simulink model "untitled"  (R2023a)
settings: Solver=VariableStepAuto  StartTime=0.0  StopTime=10.0  RelTol=1e-3
values from neighbouring files (symbols this model uses):
  e = 0    [orb_elem.m]
  mi = (mi)    [orb_elem.m]
undefined symbols (not defined in the file or in its folder): Cd0, Cd1, drag, h0_ini, i0_ini, J2, J2_dist, l0, l1, m0, m1, man, ohm0_ini, omega_E, pcoRad, r0_dot_ini, r0_ini, Re, theta0_ini, x0_dot_ini, x0_ini, y0_dot_ini, y0_ini, z0_dot_ini, z0_ini
(part 1 of 2)
settings Model: Creator=rodri  LastModifiedBy=rodri

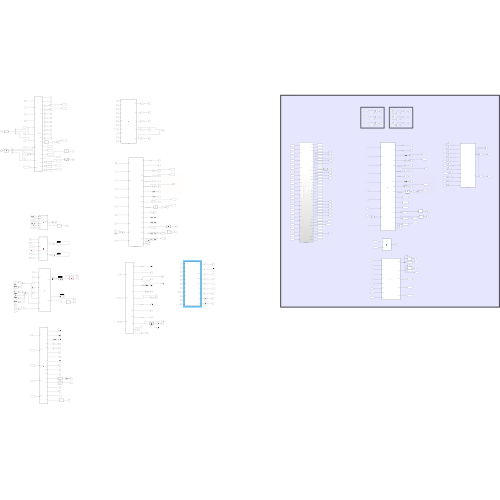
[thumbnail: Simulink's stored preview of the top-level diagram]
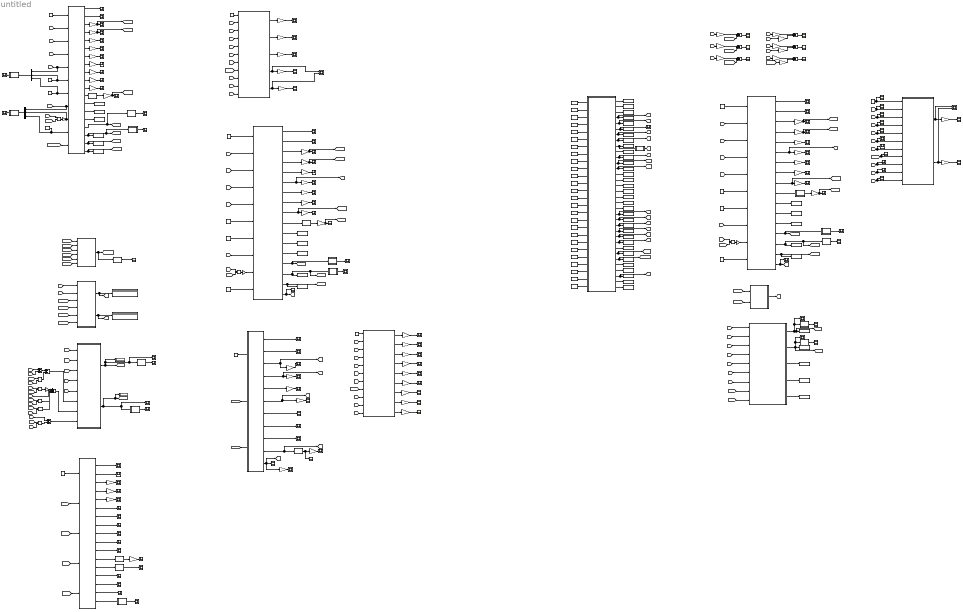
== system untitled ==
  note: Diferença elementos orbitais do líder e do seguidor
  note: Diferença elementos orbitais do líder e do seguidor
  note: Diferença elementos orbitais do líder entre o integral e o calculado
  Add : Sum
  Add1 : Sum  Inputs=+-
  Add2 : Sum  Inputs=+++-
  Add3 : Sum
  Constant{1,6,8,15,36} (5 alike) : Constant  Value=mi
  Constant{3..5,7,9..11,13..14,33,45..46} (12 alike) : Constant  Value=0
  Constant12 : Constant  Value=Re
  Constant2 : Constant  Value=Re
  Constant34 : Constant  Value=r0_dot_ini
  Constant35 : Constant  Value=Re
  Constant37 : Constant  Value=theta0_ini
  Constant41 : Constant  Value=ohm0_ini
  Constant42 : Constant  Value=e  LockScale=on
  Constant43 : Constant  Value=m1
  Constant44 : Constant  Value=J2_dist  OutDataTypeStr=boolean
  Constant47 : Constant  Value=x0_ini
  Constant48 : Constant  Value=Cd1
  Constant49 : Constant  Value=m0
  Constant50 : Constant  Value=y0_ini
  Constant51 : Constant  Value=z0_ini
  Constant52 : Constant  Value=x0_dot_ini
  Constant53 : Constant  Value=y0_dot_ini
  Constant54 : Constant  Value=z0_dot_ini
  Constant55 : Constant  Value=man
  Constant56 : Constant  Value=pcoRad
  Constant57 : Constant  Value=l1
  Constant58 : Constant  Value=l0
  Constant59 : Constant  Value=r0_ini
  Constant60 : Constant  Value=Cd0
  Constant61 : Constant  Value=drag  OutDataTypeStr=boolean
  Constant62 : Constant  Value=h0_ini
  Constant63 : Constant  Value=i0_ini
  Display{,1..3} (4 alike) : Display
  ElemOrbLider : MATLAB Function  TreatAsAtomicUnit=on
  ElemOrbLider1 : MATLAB Function  TreatAsAtomicUnit=on
  ElemOrbLider2 : MATLAB Function  TreatAsAtomicUnit=on
  Gain{,1..9,12..28,30..43,45..64} (61 alike) : Gain  Gain=180/pi
  Gain{10..11,29,44} (4 alike) : Gain
  GuiamentoOrbital1 : Subsystem
  MATLAB Function : MATLAB Function  TreatAsAtomicUnit=on
  MATLAB Function1 : MATLAB Function  TreatAsAtomicUnit=on
  MATLAB Function10 : MATLAB Function  TreatAsAtomicUnit=on
  MATLAB Function11 : MATLAB Function  TreatAsAtomicUnit=on
  MATLAB Function12 : MATLAB Function  TreatAsAtomicUnit=on
  MATLAB Function13 : MATLAB Function  TreatAsAtomicUnit=on
  MATLAB Function14 : MATLAB Function  TreatAsAtomicUnit=on
  MATLAB Function15 : MATLAB Function  TreatAsAtomicUnit=on
  MATLAB Function16 : MATLAB Function  TreatAsAtomicUnit=on
  MATLAB Function17 : MATLAB Function  TreatAsAtomicUnit=on
  MATLAB Function18 : MATLAB Function  TreatAsAtomicUnit=on
  MATLAB Function19 : MATLAB Function  TreatAsAtomicUnit=on
  MATLAB Function2 : MATLAB Function  TreatAsAtomicUnit=on
  MATLAB Function3 : MATLAB Function  TreatAsAtomicUnit=on
  MATLAB Function4 : MATLAB Function  TreatAsAtomicUnit=on
  MATLAB Function5 : MATLAB Function  TreatAsAtomicUnit=on
  MATLAB Function6 : MATLAB Function  TreatAsAtomicUnit=on
  MATLAB Function7 : MATLAB Function  TreatAsAtomicUnit=on
  MATLAB Function8 : MATLAB Function  TreatAsAtomicUnit=on
  MATLAB Function9 : MATLAB Function  TreatAsAtomicUnit=on
  Minus{,1..5} (6 alike) : Sum  Inputs=+-
  Mux2 : Mux  Inputs=3
  Mux3 : Mux  Inputs=3
  Nadir1 : MATLAB Function  TreatAsAtomicUnit=on
  Nadir2 : MATLAB Function  TreatAsAtomicUnit=on
  Nadir3 : MATLAB Function  TreatAsAtomicUnit=on
  OrbEleSeg : MATLAB Function  TreatAsAtomicUnit=on
  OrbEleSeg1 : MATLAB Function  TreatAsAtomicUnit=on
  Product{,1..7} (8 alike) : Product
  Scope{,1..74,76..103,105..116} (115 alike) : Scope
  Scope104 : Scope  NumInputPorts=2
  Scope75 : Scope  NumInputPorts=2
  To Workspace1 : ToWorkspace  VariableName=r0x_vec_I1  SaveFormat=Timeseries  SampleTime=-1
  To Workspace10 : ToWorkspace  VariableName=h0_vec_I2  SaveFormat=Timeseries  SampleTime=-1
  To Workspace11 : ToWorkspace  VariableName=r0x_vec_I2  SaveFormat=Timeseries  SampleTime=-1
  To Workspace12 : ToWorkspace  VariableName=v0_vec_I2  SaveFormat=Timeseries  SampleTime=-1
  To Workspace13 : ToWorkspace  VariableName=r0y_vec_I2  SaveFormat=Timeseries  SampleTime=-1
  To Workspace14 : ToWorkspace  VariableName=v1_vec_I  SaveFormat=Timeseries  SampleTime=-1
  To Workspace15 : ToWorkspace  VariableName=r1x_vec_I  SaveFormat=Timeseries  SampleTime=-1
  To Workspace16 : ToWorkspace  VariableName=r1y_vec_I  SaveFormat=Timeseries  SampleTime=-1
  To Workspace17 : ToWorkspace  VariableName=r1z_vec_I  SaveFormat=Timeseries  SampleTime=-1
  To Workspace18 : ToWorkspace  VariableName=r0z_vec_I2  SaveFormat=Timeseries  SampleTime=-1
  To Workspace2 : ToWorkspace  VariableName=r0x_vec_I  SaveFormat=Timeseries  SampleTime=-1
  To Workspace28 : ToWorkspace  VariableName=v0_vec_I  SaveFormat=Timeseries  SampleTime=-1
  To Workspace3 : ToWorkspace  VariableName=r0y_vec_I  SaveFormat=Timeseries  SampleTime=-1
  To Workspace34 : ToWorkspace  VariableName=x_dotdot  SaveFormat=Timeseries  SampleTime=-1
  To Workspace35 : ToWorkspace  VariableName=y_dotdot  SaveFormat=Timeseries  SampleTime=-1
  To Workspace36 : ToWorkspace  VariableName=ohm0  SaveFormat=Timeseries  SampleTime=-1
  To Workspace37 : ToWorkspace  VariableName=omega_x  SaveFormat=Timeseries  SampleTime=-1
  To Workspace38 : ToWorkspace  VariableName=omega_z  SaveFormat=Timeseries  SampleTime=-1
  To Workspace39 : ToWorkspace  VariableName=dx0  SaveFormat=Timeseries  SampleTime=-1
  To Workspace4 : ToWorkspace  VariableName=r0z_vec_I  SaveFormat=Timeseries  SampleTime=-1
  To Workspace40 : ToWorkspace  VariableName=dy0  SaveFormat=Timeseries  SampleTime=-1
  To Workspace41 : ToWorkspace  VariableName=dz0  SaveFormat=Timeseries  SampleTime=-1
  To Workspace45 : ToWorkspace  VariableName=a0_vec_I  SaveFormat=Timeseries  SampleTime=-1
  To Workspace46 : ToWorkspace  VariableName=h0_vec_I  SaveFormat=Timeseries  SampleTime=-1
  To Workspace47 : ToWorkspace  VariableName=delta_Dx  SaveFormat=Timeseries  SampleTime=-1
  To Workspace48 : ToWorkspace  VariableName=delta_Dy  SaveFormat=Timeseries  SampleTime=-1
  To Workspace49 : ToWorkspace  VariableName=delta_Dz  SaveFormat=Timeseries  SampleTime=-1
  To Workspace5 : ToWorkspace  VariableName=v0_vec_I1  SaveFormat=Timeseries  SampleTime=-1
  To Workspace50 : ToWorkspace  VariableName=rho_a0  SaveFormat=Timeseries  SampleTime=-1
  To Workspace51 : ToWorkspace  VariableName=z_dotdot  SaveFormat=Timeseries  SampleTime=-1
  To Workspace52 : ToWorkspace  VariableName=x  SaveFormat=Timeseries  SampleTime=-1
  To Workspace53 : ToWorkspace  VariableName=x_dot  SaveFormat=Timeseries  SampleTime=-1
  To Workspace54 : ToWorkspace  VariableName=y  SaveFormat=Timeseries  SampleTime=-1
  To Workspace55 : ToWorkspace  VariableName=y_dot  SaveFormat=Timeseries  SampleTime=-1
  To Workspace56 : ToWorkspace  VariableName=z  SaveFormat=Timeseries  SampleTime=-1
  To Workspace57 : ToWorkspace  VariableName=z_dot  SaveFormat=Timeseries  SampleTime=-1
  To Workspace58 : ToWorkspace  VariableName=rho_a1  SaveFormat=Timeseries  SampleTime=-1
  To Workspace59 : ToWorkspace  VariableName=r0_dotdot  SaveFormat=Timeseries  SampleTime=-1
  To Workspace6 : ToWorkspace  VariableName=r0y_vec_I1  SaveFormat=Timeseries  SampleTime=-1
  To Workspace60 : ToWorkspace  VariableName=omega_z_dot  SaveFormat=Timeseries  SampleTime=-1
  To Workspace61 : ToWorkspace  VariableName=dx1  SaveFormat=Timeseries  SampleTime=-1
  To Workspace62 : ToWorkspace  VariableName=r0  SaveFormat=Timeseries  SampleTime=-1
  To Workspace63 : ToWorkspace  VariableName=dy1  SaveFormat=Timeseries  SampleTime=-1
  To Workspace64 : ToWorkspace  VariableName=dz1  SaveFormat=Timeseries  SampleTime=-1
  To Workspace65 : ToWorkspace  VariableName=omega_y_dot  SaveFormat=Timeseries  SampleTime=-1
  To Workspace66 : ToWorkspace  VariableName=omega_x_dot  SaveFormat=Timeseries  SampleTime=-1
  To Workspace67 : ToWorkspace  VariableName=h0  SaveFormat=Timeseries  SampleTime=-1
  To Workspace68 : ToWorkspace  VariableName=r1  SaveFormat=Timeseries  SampleTime=-1
  To Workspace69 : ToWorkspace  VariableName=r0_dot  SaveFormat=Timeseries  SampleTime=-1
  To Workspace7 : ToWorkspace  VariableName=r0z_vec_I1  SaveFormat=Timeseries  SampleTime=-1
  To Workspace70 : ToWorkspace  VariableName=i0  SaveFormat=Timeseries  SampleTime=-1
  To Workspace71 : ToWorkspace  VariableName=theta0  SaveFormat=Timeseries  SampleTime=-1
  To Workspace72 : ToWorkspace  VariableName=theta0_dot  SaveFormat=Timeseries  SampleTime=-1
  To Workspace8 : ToWorkspace  VariableName=h0_vec_I1  SaveFormat=Timeseries  SampleTime=-1
  To Workspace9 : ToWorkspace  VariableName=r1_vec_I  SaveFormat=Timeseries  SampleTime=-1
  wrapTo2pi1 : MATLAB Function  TreatAsAtomicUnit=on
  wrapTo2pi2 : MATLAB Function  TreatAsAtomicUnit=on
  wrapTo2pi3 : MATLAB Function  TreatAsAtomicUnit=on
  wrapTo2pi4 : MATLAB Function  TreatAsAtomicUnit=on
  wrapTo2pi5 : MATLAB Function  TreatAsAtomicUnit=on
  wrapTo2pi6 : MATLAB Function  TreatAsAtomicUnit=on
  wires:
  Product/1 -> Gain11/1
  Constant8/1 -> ElemOrbLider/1(mi)
  Gain10/1 -> Add2/1
  [v0_vec_I] -> OrbEleSeg/5(v0_vec_I)
  [z] -> Product4/2
  [x] -> Product3/2
  Add1/1 -> MATLAB Function5/6(x_dot)
  [r0_dot] -> Add/1
  ElemOrbLider/6(f1) -> Gain3/1
  Mux2/1 -> MATLAB Function14/1(u)
  Constant7/1 -> Mux2/3, ElemOrbLider/7(z)
  Add/1 -> Add1/1
  ElemOrbLider/2(e1) -> Scope1/1
  [h0_vec_I] -> MATLAB Function3/6(h0_vec_I)
  OrbEleSeg/7(u1) -> Scope63/1
  ElemOrbLider/5(omega1) -> Gain2/1
  [r0_vec_I] -> OrbEleSeg/4(r0_vec_I)
  [z] -> MATLAB Function5/5(z)
  OrbEleSeg/5(omega1) -> Gain41/1
  OrbEleSeg/17(v1_vec_I) -> MATLAB Function10/1(x)
  MATLAB Function16/1(rho) -> Scope30/1
  Gain41/1 -> Scope61/1
  MATLAB Function9/1(rho) -> Scope78/1
  MATLAB Function6/1(y) -> Scope72/1
  MATLAB Function8/1(rho) -> Scope77/1
  ElemOrbLider/15(r0z_I) -> To Workspace4/1
  OrbEleSeg/4(Ohm1) -> Gain40/1
  [h0] -> MATLAB Function3/2(h0)
  OrbEleSeg/10(omega_t1) -> Scope66/1
  OrbEleSeg/3(i1) -> Gain39/1
  [rho_vec_I] -> OrbEleSeg/2(rho_vec_I)
  Gain40/1 -> Scope60/1
  Gain42/1 -> Scope68/1
  Constant36/1 -> OrbEleSeg/1(mi)
  [y] -> MATLAB Function5/4(y)
  [omega_z] -> MATLAB Function/2(omega_z)
  [r0_dotdot_vec] -> ElemOrbLider/11(r0_dotdot_vec)
  Gain39/1 -> Scope59/1
  OrbEleSeg/11(lambda1) -> Scope67/1
  OrbEleSeg/12(theta1) -> wrapTo2pi3/1(u)
  [omega_z_dot] -> MATLAB Function/4(omega_z_dot)
  MATLAB Function14/1(y) -> Scope24/1
  [omega_x] -> MATLAB Function/6(omega_x)
  [a0_vec_I] -> MATLAB Function3/5(a0_vec_I)
  [omega_x] -> Product4/1
  ElemOrbLider/19(h0_vec_I) -> [h0_vec_I], To Workspace46/1
  wrapTo2pi3/1(y) -> Gain42/1
  [C_dot] -> MATLAB Function5/2(C_dot)
  [C] -> MATLAB Function5/1(C)
  ElemOrbLider/18(a0_vec_I) -> [a0_vec_I], To Workspace45/1
  [r0_dot] -> MATLAB Function/5(r0_dot)
  Gain4/1 -> [theta0_calc], Scope6/1
  [r0_dotdot] -> MATLAB Function/1(r0_dotdot)
  OrbEleSeg/8(L1) -> Scope64/1
  ElemOrbLider/11(lambda1) -> Gain9/1
  [ohm0] -> ElemOrbLider/2(ohm)
  Gain3/1 -> Scope5/1
  ElemOrbLider/3(i1) -> Gain/1
  Gain2/1 -> Scope4/1
  Gain/1 -> [i0_calc], Scope2/1
  Gain5/1 -> Scope7/1
  Gain6/1 -> Scope8/1
  [theta0] -> ElemOrbLider/3(theta)
  ElemOrbLider/12(theta1) -> wrapTo2pi2/1(u)
  [r0] -> Product/1
  ElemOrbLider/8(L1) -> Gain6/1
  ElemOrbLider/16(r0_vec_I) -> MATLAB Function7/1(x), [r0_vec_I]
  ElemOrbLider/1(a1) -> Scope/1
  Product4/1 -> Add2/4
  [omega_z] -> Product3/1
  ElemOrbLider/13(r0x_I) -> To Workspace2/1
  MATLAB Function3/2(C_dot) -> [C_dot], Display1/1
  OrbEleSeg/2(e1) -> Scope58/1
  [r0] -> MATLAB Function3/1(r0)
  Product1/1 -> Add1/2
  [r0_dot] -> Mux3/1, ElemOrbLider/8(x_dot)
  MATLAB Function15/1(y) -> Scope25/1
  [x_dot] -> Add/2
  OrbEleSeg/9(l1) -> Scope65/1
  [y] -> Product5/2
  Product5/1 -> Add3/2
  ElemOrbLider/17(v0_vec_I) -> MATLAB Function8/1(x), [v0_vec_I], To Workspace28/1
  ElemOrbLider/7(u1) -> Gain5/1
  [omega_z] -> Product1/1
  Gain7/1 -> Scope9/1
  OrbEleSeg/16(r1z_I) -> Scope12/1
  [omega_z] -> Product2/2
  [y_dot] -> Add2/2
  ElemOrbLider/9(l1) -> Gain7/1
  OrbEleSeg/1(a1) -> Scope57/1
  Constant9/1 -> ElemOrbLider/10(z_dot), Mux3/3
  Gain11/1 -> Mux3/2, ElemOrbLider/9(y_dot)
  [x] -> MATLAB Function5/3(x)
  MATLAB Function5/2(rho_dot_vec_I) -> [rho_dot_vec_I], Display3/1, Scope27/1, MATLAB Function16/1(x)
  MATLAB Function3/1(C) -> Display/1, [C]
  ElemOrbLider/14(r0y_I) -> To Workspace3/1
  ElemOrbLider/10(omega_t1) -> Gain8/1
  MATLAB Function5/1(rho_vec_I) -> Scope26/1, MATLAB Function17/1(x), Display2/1, [rho_vec_I]
  ElemOrbLider/4(Ohm1) -> Gain1/1
  [z_dot] -> Add3/1
  [i0] -> ElemOrbLider/4(I)
  Product2/1 -> Gain10/1
  MATLAB Function17/1(rho) -> Scope29/1
  [r0] -> Product2/1
  wrapTo2pi2/1(y) -> Gain4/1
  OrbEleSeg/13(r1_vec_I) -> MATLAB Function9/1(x)
  [r0] -> MATLAB Function/3(r0)
  [omega_z] -> Product/2
  OrbEleSeg/14(r1x_I) -> Scope14/1
  MATLAB Function/1(r0_dotdot_vec) -> MATLAB Function6/1(u), [r0_dotdot_vec]
  OrbEleSeg/15(r1y_I) -> Scope13/1
  [omega_x] -> Product5/1
  Gain9/1 -> Scope11/1
  [rho_dot_vec_I] -> OrbEleSeg/3(rho_dot_vec_I)
  [y] -> Product1/2
  Add3/1 -> MATLAB Function5/8(z_dot)
  Mux3/1 -> MATLAB Function15/1(u)
  Constant5/1 -> Mux2/2, ElemOrbLider/6(y)
  OrbEleSeg/6(f1) -> Scope62/1
  MATLAB Function10/1(rho) -> Scope79/1
  Gain1/1 -> [ohm0_calc], Scope3/1
  MATLAB Function7/1(rho) -> Scope76/1
  [r0_vec_I] -> MATLAB Function3/3(r0_vec_I)
  Add2/1 -> MATLAB Function5/7(y_dot)
  Product3/1 -> Add2/3
  [r0] -> Mux2/1, ElemOrbLider/5(x)
  Gain8/1 -> Scope10/1
  [v0_vec_I] -> MATLAB Function3/4(v0_vec_I)
  Gain50/1 -> Scope44/1
  [i0] -> Nadir2/7(i0)
  [ohm1] -> Nadir2/9(ohm1)
  [y] -> Nadir2/4(y)
  Constant35/1 -> Nadir2/1(Re)
  Gain51/1 -> Scope42/1
  [z] -> Nadir2/5(z)
  [ohm0] -> Nadir2/6(ohm0)
  [r0] -> Nadir2/2(r0)
  Nadir2/4(PHI) -> Scope75/1, Gain52/1
  Gain53/1 -> Scope74/1
  [i1] -> Nadir2/10(i1)
  Gain52/1 -> Scope73/1
  Nadir2/3(LF1) -> Gain51/1
  [x] -> Nadir2/3(x)
  [L0] -> Nadir2/8(f0)
  [L1] -> Nadir2/11(f1)
  Nadir2/5(THETA) -> Scope75/2, Gain53/1
  Nadir2/2(psi_ref) -> Gain50/1  "psi_ref"
  Nadir2/1(phi_ref) -> Gain49/1  "phi_ref"
  Gain49/1 -> Scope43/1
  Nadir1/3(alpha_F1) -> Gain12/1
  OrbEleSeg1/6(f1) -> [f1], Gain25/1  "Anomalia verdadeira"
  wrapTo2pi4/1(y) -> Scope16/1, Gain16/1
  Gain21/1 -> Scope32/1
  Gain18/1 -> Scope21/1
  Gain17/1 -> Scope20/1
  OrbEleSeg1/4(Ohm1) -> [ohm1], Gain14/1  "Longitude do nodo ascendente"
  Nadir1/1(LF1) -> Gain24/1
  OrbEleSeg1/10(theta1) -> [theta1], wrapTo2pi4/1(u)  "Argumento de latitude"
  [z] -> Nadir1/5(z)
  Gain13/1 -> Scope34/1
  Nadir1/5(alpha_f) -> Gain18/1
  [ohm0] -> Nadir1/6(ohm0)
  OrbEleSeg1/9(lambda1) -> Scope40/1  "Longitude média"
  Gain14/1 -> Scope36/1
  OrbEleSeg1/3(i1) -> [i1], Gain13/1  "inclinação"
  OrbEleSeg1/2(e1) -> Scope23/1  "excentricidade"
  Gain15/1 -> Scope37/1
  Gain22/1 -> Scope33/1
  Nadir1/8(psi_ref) -> Gain21/1
  Gain16/1 -> Scope41/1
  Gain19/1 -> Scope28/1
  OrbEleSeg1/1(a1) -> Scope22/1  "semi-eixo maior"
  OrbEleSeg1/7(l1) -> Scope38/1  "Latitude média"
  [i0] -> Nadir1/7(i0)
  Constant1/1 -> OrbEleSeg1/1(mi)
  [L1] -> Nadir1/8(L0)
  Constant2/1 -> Nadir1/1(Re)
  [v1_vec_I] -> OrbEleSeg1/3(v1_vec_I)
  [L1] -> Nadir1/11(L1)
  Nadir1/9(phi_ref) -> Gain22/1
  Nadir1/7(THETA) -> Gain20/1
  [ohm1] -> Nadir1/9(ohm1)
  Gain12/1 -> Scope19/1
  OrbEleSeg1/8(omega_t1) -> Scope39/1  "Longitude do pericentro"
  [i1] -> Nadir1/10(i1)
  [x] -> Nadir1/3(x)
  [r0] -> Nadir1/2(r0)
  Gain23/1 -> Scope35/1
  Gain26/1 -> Scope18/1
  [y] -> Nadir1/4(y)
  Gain24/1 -> Scope45/1
  Nadir1/6(PHI) -> Gain19/1
  OrbEleSeg1/11(L1) -> [L1], Gain26/1, Scope17/1
  Nadir1/2(LF2) -> Gain23/1
  [r1_vec_I] -> OrbEleSeg1/2(r1_vec_I)
  OrbEleSeg1/5(omega1) -> Gain15/1  "Argumento do pericentro"
  Gain25/1 -> Scope15/1
  Gain20/1 -> Scope31/1
  Nadir1/4(alpha_F2) -> Gain17/1
  [theta0] -> ElemOrbLider1/3(theta)
  ElemOrbLider1/3(i0) -> Gain27/1  "inclinação"
  ElemOrbLider1/15(v0_vec_I) -> To Workspace5/1, MATLAB Function2/1(x), [v0_vec_I]
  Product6/1 -> Gain29/1
  Constant10/1 -> ElemOrbLider1/10(z_dot)
  Constant4/1 -> ElemOrbLider1/7(z)
  ElemOrbLider1/2(e0) -> Scope47/1  "excentricidade"
  Gain30/1 -> Scope51/1
  Gain35/1 -> Scope70/1
  [r0] -> Product6/1
  [ohm0] -> ElemOrbLider1/2(ohm)
  ElemOrbLider1/1(a0) -> Scope46/1  "semi-eixo maior"
  ElemOrbLider1/5(omega0) -> Gain30/1  "Argumento do pericentro"
  Gain32/1 -> [theta0_calc], Scope53/1
  Gain34/1 -> Scope69/1
  ElemOrbLider1/9(lambda0) -> [lambda0], Gain35/1  "Longitude média"
  Gain31/1 -> Scope52/1
  [r0_dot] -> ElemOrbLider1/8(x_dot)
  ElemOrbLider1/12(r0y_I) -> To Workspace6/1
  [omega_z] -> Product6/2
  MATLAB Function2/1(rho) -> Scope56/1
  ElemOrbLider1/10(theta0) -> wrapTo2pi1/1(u)  "Argumento de latitude"
  ElemOrbLider1/6(f0) -> [f0], Gain31/1  "Anomalia verdadeira"
  ElemOrbLider1/16(h0_vec_I) -> To Workspace8/1, [h0_vec_I]
  wrapTo2pi1/1(y) -> Gain32/1
  Gain33/1 -> Scope54/1
  MATLAB Function1/1(rho) -> Scope55/1
  Gain29/1 -> ElemOrbLider1/9(y_dot)
  ElemOrbLider1/4(Ohm0) -> Gain28/1  "Longitude do nodo ascendente"
  ElemOrbLider1/13(r0z_I) -> To Workspace7/1
  Gain28/1 -> [ohm0_calc], Scope50/1
  Constant6/1 -> ElemOrbLider1/1(mi)
  ElemOrbLider1/17(L0) -> [L0], Scope48/1
  ElemOrbLider1/14(r0_vec_I) -> [r0_vec_I], MATLAB Function1/1(x)
  ElemOrbLider1/7(l0) -> Gain33/1  "Latitude média"
  Gain27/1 -> [i0_calc], Scope49/1
  ElemOrbLider1/8(omega_t0) -> Gain34/1  "Longitude do perigeu"
  Constant3/1 -> ElemOrbLider1/6(y)
  [i0] -> ElemOrbLider1/4(I)
  ElemOrbLider1/11(r0x_I) -> To Workspace1/1
  [r0] -> ElemOrbLider1/5(x)
  [r0] -> Scope90/1, Nadir3/2(r0)  "r0"
  Constant60/1 -> GuiamentoOrbital1/3(Cd0)
  GuiamentoOrbital1/18(delta_Dy) -> To Workspace48/1
  Minus/1 -> Scope108/1
  [y] -> Scope92/1, Nadir3/4(y)  "y"
  GuiamentoOrbital1/16(dz0) -> To Workspace41/1
  [i1] -> Scope101/1, Nadir3/10(i1)  "i1"
  MATLAB Function11/1(y) -> Scope84/1
  [i0] -> Scope96/1, Nadir3/7(i0)  "i0"
  GuiamentoOrbital1/31(dy1) -> To Workspace63/1
  [z] -> Scope94/1, Nadir3/5(z)  "z"
  Nadir3/1(AZ) -> Scope104/1, Gain46/1  "AZ"
  [ohm0] -> Scope95/1, Nadir3/6(ohm0)  "ohm0"
  Minus5/1 -> Scope114/1
  [x] -> Scope91/1, Nadir3/3(x)  "x"
  [L0] -> Scope99/1, Nadir3/8(L0)  "L0"
  Nadir3/2(EL) -> Scope104/2, Gain45/1  "EL"
  Minus2/1 -> Scope109/1
  MATLAB Function4/2(v1_vec_I) -> [v1_vec_I], Scope83/1, MATLAB Function13/1(u), To Workspace14/1
  [ohm1] -> Scope100/1, Nadir3/9(ohm1)  "ohm1"
  [r0_vec_I] -> MATLAB Function4/8(r0_vec_I)
  Constant48/1 -> GuiamentoOrbital1/5(Cd1)
  Constant53/1 -> GuiamentoOrbital1/17(y0_dot_ini)
  Constant52/1 -> GuiamentoOrbital1/16(x0_dot_ini)
  Gain46/1 -> Scope98/1
  MATLAB Function4/3(r1x_vec_I) -> To Workspace15/1
  MATLAB Function13/1(y) -> Scope85/1
  GuiamentoOrbital1/27(rho_a1) -> To Workspace58/1
  Constant41/1 -> GuiamentoOrbital1/12(ohm0_ini)
  wrapTo2pi5/1(y) -> [theta0]
  Constant44/1 -> GuiamentoOrbital1/23(J2_dist)
  [z_dot] -> MATLAB Function4/7(z_dot)
  Constant58/1 -> GuiamentoOrbital1/2(l0)
  [C] -> MATLAB Function4/1(C)
  [x] -> MATLAB Function4/2(x)
  Minus3/1 -> Scope113/1
  [z] -> MATLAB Function4/4(z)
  [i1] -> Gain62/1
  [v0_vec_I] -> MATLAB Function4/9(v0_vec_I)
  [x_dot] -> MATLAB Function4/5(x_dot)
  [y_dot] -> MATLAB Function4/6(y_dot)
  Constant61/1 -> GuiamentoOrbital1/21(drag)
  GuiamentoOrbital1/6(r1) -> Scope89/1, To Workspace68/1
  [theta1] -> Gain64/1
  Constant47/1 -> GuiamentoOrbital1/13(x0_ini)
  Gain45/1 -> Scope97/1
  GuiamentoOrbital1/20(rho_a0) -> To Workspace50/1
  Constant54/1 -> GuiamentoOrbital1/18(z0_dot_ini)
  Constant59/1 -> GuiamentoOrbital1/8(r0_ini)
  GuiamentoOrbital1/19(delta_Dz) -> To Workspace49/1
  Constant56/1 -> GuiamentoOrbital1/20(pcoRad)
  Gain59/1 -> Minus3/1
  [ohm0] -> Gain60/1
  Gain57/1 -> Minus1/1
  GuiamentoOrbital1/11(ohm0) -> [ohm0], To Workspace36/1
  [theta0] -> Gain61/1
  Gain62/1 -> Minus3/2
  Gain58/1 -> Minus2/1
  MATLAB Function12/1(C) -> [C]
  [i0] -> Gain59/1
  [r0_vec_I] -> MATLAB Function12/1(r0_vec_I)
  [h0_vec_I] -> MATLAB Function12/2(h0_vec_I)
  Gain64/1 -> Minus5/2
  Gain61/1 -> Minus5/1
  Minus1/1 -> Scope107/1
  [i0_calc] -> Minus/2
  [ohm0_calc] -> Minus1/2
  GuiamentoOrbital1/8(i0) -> [i0], To Workspace70/1
  Constant55/1 -> GuiamentoOrbital1/19(man)
  GuiamentoOrbital1/24(y_dot) -> [y_dot], To Workspace55/1
  [y] -> MATLAB Function4/3(y)
  MATLAB Function4/5(r1z_vec_I) -> To Workspace17/1
  Constant43/1 -> GuiamentoOrbital1/4(m1)
  GuiamentoOrbital1/21(x) -> [x], To Workspace52/1
  GuiamentoOrbital1/30(dx1) -> To Workspace61/1
  GuiamentoOrbital1/10(theta0_dot) -> To Workspace72/1
  Minus4/1 -> Scope111/1
  Constant45/1 -> GuiamentoOrbital1/25(uy)
  GuiamentoOrbital1/13(omega_z) -> [omega_z], To Workspace38/1
  Constant57/1 -> GuiamentoOrbital1/6(l1)
  Constant46/1 -> GuiamentoOrbital1/26(uz)
  GuiamentoOrbital1/3(z_dotdot) -> To Workspace51/1
  GuiamentoOrbital1/28(r0_dotdot) -> [r0_dotdot], To Workspace59/1
  GuiamentoOrbital1/12(omega_x) -> [omega_x], To Workspace37/1
  [theta0] -> Gain58/1
  MATLAB Function4/4(r1y_vec_I) -> To Workspace16/1
  GuiamentoOrbital1/22(x_dot) -> [x_dot], To Workspace53/1
  Constant34/1 -> GuiamentoOrbital1/7(r0_dot_ini)
  Gain63/1 -> Minus4/2
  GuiamentoOrbital1/34(omega_x_dot) -> To Workspace66/1
  Constant50/1 -> GuiamentoOrbital1/14(y0_ini)
  Gain56/1 -> Minus/1
  GuiamentoOrbital1/26(z_dot) -> [z_dot], To Workspace57/1
  GuiamentoOrbital1/15(dy0) -> To Workspace40/1
  GuiamentoOrbital1/25(z) -> [z], To Workspace56/1
  GuiamentoOrbital1/9(theta0) -> wrapTo2pi5/1(u), To Workspace71/1
  GuiamentoOrbital1/5(h0) -> [h0], To Workspace67/1
  Constant63/1 -> GuiamentoOrbital1/10(i0_ini)
  [i0] -> Gain56/1
  GuiamentoOrbital1/32(dz1) -> [dz1], To Workspace64/1
  GuiamentoOrbital1/23(y) -> [y], To Workspace54/1
  GuiamentoOrbital1/4(r0) -> [r0], To Workspace62/1
  GuiamentoOrbital1/2(y_dotdot) -> To Workspace35/1
  GuiamentoOrbital1/33(omega_y_dot) -> To Workspace65/1
  GuiamentoOrbital1/7(r0_dot) -> [r0_dot], To Workspace69/1
  MATLAB Function4/1(r1_vec_I) -> [r1_vec_I], To Workspace9/1, Scope82/1, MATLAB Function11/1(u)
  GuiamentoOrbital1/29(omega_z_dot) -> [omega_z_dot], To Workspace60/1
  ElemOrbLider2/11(r0x_I) -> To Workspace11/1
  Constant42/1 -> GuiamentoOrbital1/22(e)
  [r0_dot] -> ElemOrbLider2/8(x_dot)
  [ohm0] -> Gain57/1
  Gain43/1 -> [ohm0_calc], Scope102/1
  [r0] -> Product7/1
  wrapTo2pi6/1(y) -> Gain47/1
  ElemOrbLider2/12(r0y_I) -> To Workspace13/1
  Gain60/1 -> Minus4/1
  ElemOrbLider2/8(omega_t0) -> Gain54/1  "Longitude do perigeu"
  Constant37/1 -> GuiamentoOrbital1/11(theta0_ini)
  [theta0] -> ElemOrbLider2/3(theta)
  Gain38/1 -> [i0_calc], Scope93/1
  Constant14/1 -> ElemOrbLider2/7(z)
  ElemOrbLider2/3(i0) -> Gain38/1  "inclinação"
  [ohm0] -> ElemOrbLider2/2(ohm)
  [L1] -> Scope103/1, Nadir3/11(L1)  "L1"
  Constant13/1 -> ElemOrbLider2/6(y)
  Gain37/1 -> Scope105/1
  ElemOrbLider2/15(v0_vec_I) -> To Workspace12/1, MATLAB Function19/1(x), [v0_vec_I]
  ElemOrbLider2/2(e0) -> Scope86/1  "excentricidade"
  Gain54/1 -> Scope80/1
  ElemOrbLider2/1(a0) -> Scope71/1  "semi-eixo maior"
  ElemOrbLider2/14(r0_vec_I) -> [r0_vec_I], MATLAB Function18/1(x)
  Constant49/1 -> GuiamentoOrbital1/1(m0)
  Gain36/1 -> Scope110/1
  Gain55/1 -> Scope81/1
  GuiamentoOrbital1/17(delta_Dx) -> To Workspace47/1
  [ohm1] -> Gain63/1
  GuiamentoOrbital1/1(x_dotdot) -> To Workspace34/1
  ElemOrbLider2/9(lambda0) -> [lambda0], Gain55/1  "Longitude média"
  ElemOrbLider2/16(h0_vec_I) -> To Workspace10/1, [h0_vec_I]
  MATLAB Function18/1(rho) -> Scope115/1
  [omega_z] -> Product7/2
  ElemOrbLider2/13(r0z_I) -> To Workspace18/1
  Constant62/1 -> GuiamentoOrbital1/9(h0_ini)
  ElemOrbLider2/7(l0) -> Gain48/1  "Latitude média"
  MATLAB Function19/1(rho) -> Scope116/1
  Product7/1 -> Gain44/1
  ElemOrbLider2/6(f0) -> [f0], Gain37/1  "Anomalia verdadeira"
  Gain44/1 -> ElemOrbLider2/9(y_dot)
  Constant12/1 -> Scope88/1, Nadir3/1(Re)  "Re"
  Gain48/1 -> Scope112/1
  Constant33/1 -> GuiamentoOrbital1/24(ux)
  Constant15/1 -> ElemOrbLider2/1(mi)
  ElemOrbLider2/4(Ohm0) -> Gain43/1  "Longitude do nodo ascendente"
  GuiamentoOrbital1/14(dx0) -> To Workspace39/1
  Constant11/1 -> ElemOrbLider2/10(z_dot)
  Constant51/1 -> GuiamentoOrbital1/15(z0_ini)
  [r0] -> ElemOrbLider2/5(x)
  Gain47/1 -> [theta0_calc], Scope106/1
  ElemOrbLider2/5(omega0) -> Gain36/1  "Argumento do pericentro"
  [i0] -> ElemOrbLider2/4(I)
  [theta0_calc] -> Minus2/2
  ElemOrbLider2/10(theta0) -> wrapTo2pi6/1(u)  "Argumento de latitude"
  ElemOrbLider2/17(L0) -> [L0], Scope87/1

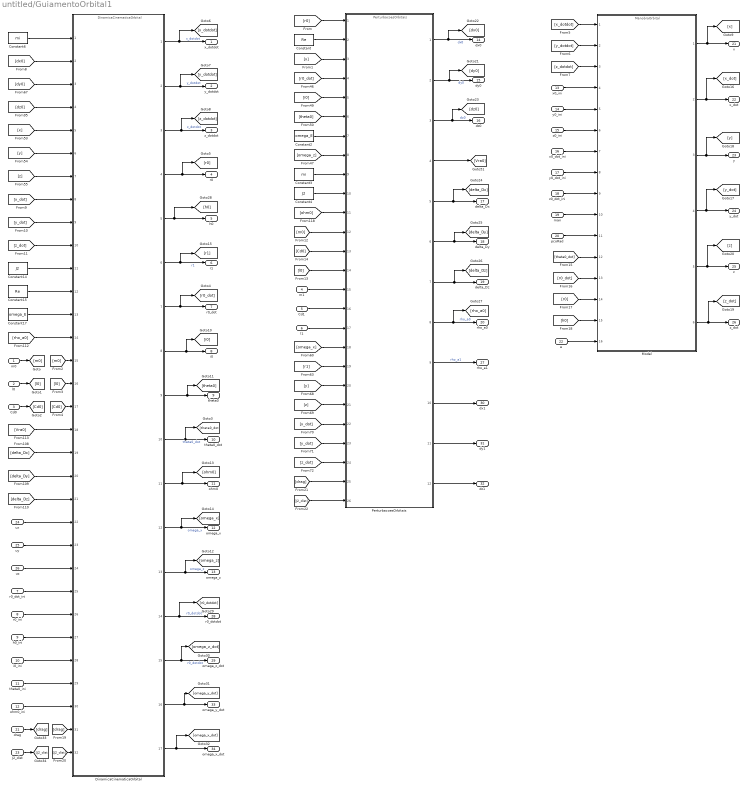
== system untitled/GuiamentoOrbital1 ==
  m0 : Inport  OutDataTypeStr=double  PortDimensions=1
  l0 : Inport  Port=2  OutDataTypeStr=double  PortDimensions=1
  Cd0 : Inport  Port=3  OutDataTypeStr=double  PortDimensions=1
  m1 : Inport  Port=4  OutDataTypeStr=double  PortDimensions=1
  Cd1 : Inport  Port=5  OutDataTypeStr=double  PortDimensions=1
  l1 : Inport  Port=6  OutDataTypeStr=double  PortDimensions=1
  r0_dot_ini : Inport  Port=7  OutDataTypeStr=double  PortDimensions=1
  r0_ini : Inport  Port=8  OutDataTypeStr=double  PortDimensions=1
  h0_ini : Inport  Port=9  OutDataTypeStr=double  PortDimensions=1
  i0_ini : Inport  Port=10  OutDataTypeStr=double  PortDimensions=1
  theta0_ini : Inport  Port=11  OutDataTypeStr=double  PortDimensions=1
  ohm0_ini : Inport  Port=12  OutDataTypeStr=double  PortDimensions=1
  x0_ini : Inport  Port=13  OutDataTypeStr=double  PortDimensions=1
  y0_ini : Inport  Port=14  OutDataTypeStr=double  PortDimensions=1
  z0_ini : Inport  Port=15  OutDataTypeStr=double  PortDimensions=1
  x0_dot_ini : Inport  Port=16  OutDataTypeStr=double  PortDimensions=1
  y0_dot_ini : Inport  Port=17  OutDataTypeStr=double  PortDimensions=1
  z0_dot_ini : Inport  Port=18  OutDataTypeStr=double  PortDimensions=1
  man : Inport  Port=19  OutDataTypeStr=boolean  PortDimensions=1
  pcoRad : Inport  Port=20  OutDataTypeStr=double  PortDimensions=1
  drag : Inport  Port=21  OutDataTypeStr=boolean  PortDimensions=1
  e : Inport  Port=22  OutDataTypeStr=double  PortDimensions=1
  J2_dist : Inport  Port=23  OutDataTypeStr=boolean  PortDimensions=1
  ux : Inport  Port=24  OutDataTypeStr=double  PortDimensions=1
  uy : Inport  Port=25  OutDataTypeStr=double  PortDimensions=1
  uz : Inport  Port=26  OutDataTypeStr=double  PortDimensions=1
  Constant : Constant  Value=Re
  Constant14 : Constant  Value=J2
  Constant15 : Constant  Value=Re
  Constant17 : Constant  Value=omega_E
  Constant2 : Constant  Value=omega_E
  Constant3 : Constant  Value=mi
  Constant4 : Constant  Value=J2
  Constant6 : Constant  Value=mi
  DinamicaCinematicaOrbital : ModelReference  ModelNameDialog=DinamicaCinematicaOrbital  ModelReferenceVersion=3.29
  Model : ModelReference  ModelNameDialog=ManobraOrbital.slx  ModelReferenceVersion=3.34
  PerturbacoesOrbitais : ModelReference  ModelNameDialog=PerturbacoesOrbitais  ModelReferenceVersion=3.14
  x_dotdot : Outport  OutDataTypeStr=double  PortDimensions=1  SampleTime=0
  y_dotdot : Outport  Port=2  OutDataTypeStr=double  PortDimensions=1  SampleTime=0
  z_dotdot : Outport  Port=3  OutDataTypeStr=double  PortDimensions=1  SampleTime=0
  r0 : Outport  Port=4  OutDataTypeStr=double  PortDimensions=1  SampleTime=0
  h0 : Outport  Port=5  OutDataTypeStr=double  PortDimensions=1  SampleTime=0
  r1 : Outport  Port=6  OutDataTypeStr=double  PortDimensions=1  SampleTime=0
  r0_dot : Outport  Port=7  OutDataTypeStr=double  PortDimensions=1  SampleTime=0
  i0 : Outport  Port=8  OutDataTypeStr=double  PortDimensions=1  SampleTime=0
  theta0 : Outport  Port=9  OutDataTypeStr=double  PortDimensions=1  SampleTime=0
  theta0_dot : Outport  Port=10  OutDataTypeStr=double  PortDimensions=1  SampleTime=0
  ohm0 : Outport  Port=11  OutDataTypeStr=double  PortDimensions=1  SampleTime=0
  omega_x : Outport  Port=12  OutDataTypeStr=double  PortDimensions=1  SampleTime=0
  omega_z : Outport  Port=13  OutDataTypeStr=double  PortDimensions=1  SampleTime=0
  dx0 : Outport  Port=14  OutDataTypeStr=double  PortDimensions=1  SampleTime=[1,0]
  dy0 : Outport  Port=15  OutDataTypeStr=double  PortDimensions=1  SampleTime=[1,0]
  dz0 : Outport  Port=16  OutDataTypeStr=double  PortDimensions=1  SampleTime=[1,0]
  delta_Dx : Outport  Port=17  OutDataTypeStr=double  PortDimensions=1  SampleTime=[1,0]
  delta_Dy : Outport  Port=18  OutDataTypeStr=double  PortDimensions=1  SampleTime=[1,0]
  delta_Dz : Outport  Port=19  OutDataTypeStr=double  PortDimensions=1  SampleTime=[1,0]
  rho_a0 : Outport  Port=20  OutDataTypeStr=double  PortDimensions=1  SampleTime=[1,0]
  x : Outport  Port=21  OutDataTypeStr=double  PortDimensions=1  SampleTime=0
  x_dot : Outport  Port=22  OutDataTypeStr=double  PortDimensions=1  SampleTime=0
  y : Outport  Port=23  OutDataTypeStr=double  PortDimensions=1  SampleTime=0
  y_dot : Outport  Port=24  OutDataTypeStr=double  PortDimensions=1  SampleTime=0
  z : Outport  Port=25  OutDataTypeStr=double  PortDimensions=1  SampleTime=0
  z_dot : Outport  Port=26  OutDataTypeStr=double  PortDimensions=1  SampleTime=0
  rho_a1 : Outport  Port=27  OutDataTypeStr=double  PortDimensions=1  SampleTime=[1,0]
  r0_dotdot : Outport  Port=28  OutDataTypeStr=double  PortDimensions=1  SampleTime=0
  omega_z_dot : Outport  Port=29  OutDataTypeStr=double  PortDimensions=1  SampleTime=0
  dx1 : Outport  Port=30  OutDataTypeStr=double  PortDimensions=1  SampleTime=[1,0]
  dy1 : Outport  Port=31  OutDataTypeStr=double  PortDimensions=1  SampleTime=[1,0]
  dz1 : Outport  Port=32  OutDataTypeStr=double  PortDimensions=1  SampleTime=[1,0]
  omega_y_dot : Outport  Port=33  OutDataTypeStr=double  PortDimensions=1  SampleTime=0
  omega_x_dot : Outport  Port=34  OutDataTypeStr=double  PortDimensions=1  SampleTime=0
  wires:
  DinamicaCinematicaOrbital/6 -> r1/1, [r1]  "r1"
  PerturbacoesOrbitais/4 -> [Vra0]
  x0_dot_ini/1 -> Model/7
  DinamicaCinematicaOrbital/8 -> i0/1, [i0]
  DinamicaCinematicaOrbital/12 -> omega_x/1, [omega_x]  "omega_x"
  man/1 -> Model/10
  DinamicaCinematicaOrbital/10 -> [theta0_dot], theta0_dot/1  "theta0_dot"
  [Cd0] -> DinamicaCinematicaOrbital/17
  uz/1 -> DinamicaCinematicaOrbital/24
  [z] -> DinamicaCinematicaOrbital/7
  [Cd0] -> PerturbacoesOrbitais/13
  e/1 -> Model/16
  PerturbacoesOrbitais/9 -> rho_a1/1  "rho_a1"
  r0_ini/1 -> DinamicaCinematicaOrbital/26
  [rho_a0] -> DinamicaCinematicaOrbital/14
  [h0] -> Model/15
  [i0] -> PerturbacoesOrbitais/5
  Cd0/1 -> [Cd0]
  uy/1 -> DinamicaCinematicaOrbital/23
  [r0] -> PerturbacoesOrbitais/1
  i0_ini/1 -> DinamicaCinematicaOrbital/28
  Constant14/1 -> DinamicaCinematicaOrbital/11
  [theta0_dot] -> Model/12
  [x_dot] -> PerturbacoesOrbitais/22
  m1/1 -> PerturbacoesOrbitais/15
  theta0_ini/1 -> DinamicaCinematicaOrbital/29
  Cd1/1 -> PerturbacoesOrbitais/16
  l0/1 -> [l0]
  l1/1 -> PerturbacoesOrbitais/17
  m0/1 -> [m0]
  [m0] -> PerturbacoesOrbitais/12
  [l0] -> DinamicaCinematicaOrbital/16
  [m0] -> DinamicaCinematicaOrbital/15
  [z_dot] -> DinamicaCinematicaOrbital/10
  [y] -> DinamicaCinematicaOrbital/6
  [dy0] -> DinamicaCinematicaOrbital/3
  [y_dot] -> DinamicaCinematicaOrbital/9
  [r0] -> Model/14
  [delta_Dz] -> DinamicaCinematicaOrbital/21
  Constant15/1 -> DinamicaCinematicaOrbital/12
  PerturbacoesOrbitais/7 -> delta_Dz/1, [delta_Dz]
  [x_dot] -> DinamicaCinematicaOrbital/8
  [dz0] -> DinamicaCinematicaOrbital/4
  [x] -> DinamicaCinematicaOrbital/5
  DinamicaCinematicaOrbital/1 -> x_dotdot/1, [x_dotdot]  "x_dotdot"
  Constant3/1 -> PerturbacoesOrbitais/9
  [dx0] -> DinamicaCinematicaOrbital/2
  PerturbacoesOrbitais/2 -> [dy0], dy0/1  "dy0"
  [delta_Dx] -> DinamicaCinematicaOrbital/19
  r0_dot_ini/1 -> DinamicaCinematicaOrbital/25
  h0_ini/1 -> DinamicaCinematicaOrbital/27
  [x] -> PerturbacoesOrbitais/3
  DinamicaCinematicaOrbital/9 -> theta0/1, [theta0]
  [z_dotdot] -> Model/3
  [z] -> PerturbacoesOrbitais/21
  [Vra0] -> DinamicaCinematicaOrbital/18
  [l0] -> PerturbacoesOrbitais/14
  [r0_dot] -> PerturbacoesOrbitais/4
  PerturbacoesOrbitais/6 -> delta_Dy/1, [delta_Dy]
  ohm0_ini/1 -> DinamicaCinematicaOrbital/30
  ux/1 -> DinamicaCinematicaOrbital/22
  PerturbacoesOrbitais/1 -> dx0/1, [dx0]  "dx0"
  Constant/1 -> PerturbacoesOrbitais/2
  Model/5 -> z/1, [z]
  [y] -> PerturbacoesOrbitais/20
  Model/4 -> y_dot/1, [y_dot]
  Constant6/1 -> DinamicaCinematicaOrbital/1
  [z_dot] -> PerturbacoesOrbitais/24
  Model/1 -> x/1, [x]
  Model/3 -> y/1, [y]
  Constant4/1 -> PerturbacoesOrbitais/10
  PerturbacoesOrbitais/3 -> dz0/1, [dz0]  "dz0"
  DinamicaCinematicaOrbital/7 -> [r0_dot], r0_dot/1
  [y_dot] -> PerturbacoesOrbitais/23
  PerturbacoesOrbitais/8 -> [rho_a0], rho_a0/1  "rho_a0"
  Constant17/1 -> DinamicaCinematicaOrbital/13
  DinamicaCinematicaOrbital/5 -> [h0], h0/1
  [ohm0] -> PerturbacoesOrbitais/11
  Constant2/1 -> PerturbacoesOrbitais/7
  DinamicaCinematicaOrbital/13 -> [omega_z], omega_z/1  "omega_z"
  DinamicaCinematicaOrbital/3 -> [z_dotdot], z_dotdot/1  "z_dotdot"
  DinamicaCinematicaOrbital/2 -> [y_dotdot], y_dotdot/1  "y_dotdot"
  DinamicaCinematicaOrbital/4 -> [r0], r0/1
  [delta_Dy] -> DinamicaCinematicaOrbital/20
  Model/6 -> z_dot/1, [z_dot]
  y0_dot_ini/1 -> Model/8
  DinamicaCinematicaOrbital/11 -> [ohm0], ohm0/1
  pcoRad/1 -> Model/11
  [omega_z] -> PerturbacoesOrbitais/8
  [theta0] -> PerturbacoesOrbitais/6
  [r0_dot] -> Model/13
  [omega_x] -> PerturbacoesOrbitais/18
  y0_ini/1 -> Model/5
  [x_dotdot] -> Model/1
  x0_ini/1 -> Model/4
  [r1] -> PerturbacoesOrbitais/19
  z0_dot_ini/1 -> Model/9
  z0_ini/1 -> Model/6
  PerturbacoesOrbitais/5 -> delta_Dx/1, [delta_Dx]
  Model/2 -> x_dot/1, [x_dot]
  [y_dotdot] -> Model/2
  DinamicaCinematicaOrbital/14 -> r0_dotdot/1, [r0_dotdot]  "r0_dotdot"
  DinamicaCinematicaOrbital/15 -> omega_z_dot/1, [omega_z_dot]  "r0_dotdot"
  PerturbacoesOrbitais/10 -> dx1/1
  PerturbacoesOrbitais/11 -> dy1/1
  PerturbacoesOrbitais/12 -> dz1/1
  DinamicaCinematicaOrbital/16 -> omega_y_dot/1, [omega_y_dot]
  DinamicaCinematicaOrbital/17 -> omega_x_dot/1, [omega_x_dot]
  drag/1 -> [drag]
  J2_dist/1 -> [J2_dist]
  [drag] -> DinamicaCinematicaOrbital/31
  [J2_dist] -> DinamicaCinematicaOrbital/32
  [drag] -> PerturbacoesOrbitais/25
  [J2_dist] -> PerturbacoesOrbitais/26

== matlab function untitled/MATLAB Function1 ==
  data: x input; rho output
function rho = fcn(x)

X = x(1);
Y = x(2);
Z = x(3);

rho = sqrt(X^2+Y^2+Z^2);

== matlab function untitled/OrbEleSeg1 ==
  data: mi input; a1 output; r1_vec_I input; e1 output; i1 output; Ohm1 output; omega1 output; f1 output; l1 output; omega_t1 output; lambda1 output; theta1 output; v1_vec_I input; L1 output
function [a1,e1,i1,Ohm1,omega1,f1,l1,omega_t1,lambda1,theta1,L1] = fcn(mi,r1_vec_I,v1_vec_I)



[a1,e1,i1,Ohm1,omega1,f1,l1,omega_t1,lambda1,theta1,~,~] = orb_elem(mi,r1_vec_I',v1_vec_I');

L1 = wrapTo2Pi(omega1 + Ohm1 + f1);
%L1 = omega1 + Ohm1 + f1;

== matlab function untitled/MATLAB Function2 ==
  data: x input; rho output
function rho = fcn(x)

X = x(1);
Y = x(2);
Z = x(3);

rho = sqrt(X^2+Y^2+Z^2);

== matlab function untitled/Nadir2 ==
  data: Re input; phi_ref output; psi_ref output; r0 input; x input; y input; z input; ohm0 input; i0 input; f0 input; ohm1 input; i1 input; f1 input; LF1 output; PHI output; THETA output
function [phi_ref,psi_ref,LF1,PHI,THETA] = fcn(Re,r0,x,y,z,ohm0,i0,f0,ohm1,i1,f1)

ohm_f = ohm1;
i_f = i1;
ohm_l = ohm0;
i_l = i0;
u0_l = f0;
u0_f = f1;


% Ângulos alpha_f e alpha_l

LF1 = asin(sin(u0_f*sin(i_f)));

if u0_f >=0 && u0_f < pi
    %alpha_F1 = real(acos(complex(cos(u0_f)/cos(LF1))));
    alpha_F1 = (acos((cos(u0_f)/cos(LF1))));
else
    %alpha_F1 = 2*pi - real(acos(complex(cos(u0_f)/cos(LF1))));
    alpha_F1 = 2*pi - (acos((cos(u0_f)/cos(LF1))));
end

alpha_F2 = alpha_F1 + ohm_f;
LF2 = atan(sin(alpha_F2)*tan(i_l));

if u0_f >=0 && u0_f < pi
    alpha_f = acos(cos(LF2)*cos(alpha_F2));
else
    alpha_f = 2*pi - acos(cos(LF2)*cos(alpha_F2));
end

alpha_l = u0_l;

PHI = LF1 - LF2;
THETA = alpha_l - alpha_f;

%% EL (psi)

[~,~,R3_Ohm_l_neg] = transfer(-ohm_l);
[R1_i_l_neg,~,~] = transfer(-i_l);
[~,~,R3_alpha_f_neg] = transfer(-alpha_f);
OA = R3_Ohm_l_neg*R1_i_l_neg*R3_alpha_f_neg*[Re; 0; 0];

[~,~,R3_alpha_l_neg] = transfer(-alpha_l);
FO = -R3_Ohm_l_neg*R1_i_l_neg*R3_alpha_l_neg*[r0+x; y; z];

FA = FO + OA;

if alpha_f >= 0 && alpha_f < pi
    EL = -acos((dot(FA,FO))/(norm(FA)*norm(FO)));
else
    EL = acos((dot(FA,FO))/(norm(FA)*norm(FO)));
end

psi_ref = EL;

%% AZ (phi)

ONL = R3_Ohm_l_neg*R1_i_l_neg*R3_alpha_l_neg*[Re; 0; 0];

FNL = FO + ONL;

AZ = acos((dot(FA,FNL))/(norm(FA)*norm(FNL)));

phi_ref = AZ;

%% Cálculo das matrizes de transferência
    function [T1,T2,T3] = transfer(alpha)
        T1 = [1 0 0; 0 cos(alpha) sin(alpha); 0 -sin(alpha) cos(alpha)];
        T2 = [cos(alpha) 0 -sin(alpha); 0 1 0; sin(alpha) 0 cos(alpha)];
        T3 = [cos(alpha) sin(alpha) 0; -sin(alpha) cos(alpha) 0; 0 0 1];
    end

end

== matlab function untitled/wrapTo2pi1 ==
  data: u input; y output
function y = fcn(u)

y = wrapTo2Pi(u);

== matlab function untitled/wrapTo2pi2 ==
  data: u input; y output
function y = fcn(u)

y = wrapTo2Pi(u);

== matlab function untitled/MATLAB Function ==
  data: r0_dotdot input; r0_dotdot_vec output; omega_z input; r0 input; omega_z_dot input; r0_dot input; omega_x input
function r0_dotdot_vec = fcn(r0_dotdot,omega_z,r0,omega_z_dot,r0_dot,omega_x)

r0_dotdot_vec = [r0_dotdot-omega_z^2*r0 omega_z_dot*r0+2*omega_z*r0_dot omega_x*omega_z*r0];

== matlab function untitled/MATLAB Function3 ==
  data: r0 input; h0 input; C output; r0_vec_I input; v0_vec_I input; a0_vec_I input; h0_vec_I input; C_dot output
function [C,C_dot] = fcn(r0,h0,r0_vec_I,v0_vec_I,a0_vec_I,h0_vec_I)

r0_vec_I_uni = r0_vec_I/norm(r0_vec_I);
h0_dot_I_vec = cross(r0_vec_I,a0_vec_I);
h0_vec_I_uni = h0_vec_I/norm(h0_vec_I);


ex_vec_uni = r0_vec_I_uni;
ez_vec_uni = h0_vec_I_uni;
ey_vec_uni = cross(ez_vec_uni,ex_vec_uni);

ex_dot_vec_uni = (1/r0)*(v0_vec_I - (dot(r0_vec_I_uni,v0_vec_I)*r0_vec_I_uni));
ez_dot_vec_uni = (1/h0)*(h0_dot_I_vec - (dot(h0_vec_I_uni,h0_dot_I_vec))*h0_vec_I_uni);
ey_dot_vec_uni = cross(ex_dot_vec_uni,ez_vec_uni) + cross(ex_vec_uni,ez_dot_vec_uni);

C = [ex_vec_uni(1) ex_vec_uni(2) ex_vec_uni(3)
    ey_vec_uni(1) ey_vec_uni(2) ey_vec_uni(3)
    ez_vec_uni(1) ez_vec_uni(2) ez_vec_uni(3)];

C_dot = [ex_dot_vec_uni(1) ex_dot_vec_uni(2) ex_dot_vec_uni(3)
    ey_dot_vec_uni(1) ey_dot_vec_uni(2) ey_dot_vec_uni(3)
    ez_dot_vec_uni(1) ez_dot_vec_uni(2) ez_dot_vec_uni(3)];

== matlab function untitled/MATLAB Function5 ==
  data: C input; rho_vec_I output; C_dot input; x input; y input; z input; x_dot input; y_dot input; z_dot input; rho_dot_vec_I output
function [rho_vec_I,rho_dot_vec_I] = fcn(C,C_dot,x,y,z,x_dot,y_dot,z_dot)

rho_vec_I = C'*[x y z]';

rho_dot_vec_I = C_dot'*[x y z]' + C_dot'*[x_dot y_dot z_dot]';

== matlab function untitled/OrbEleSeg ==
  data: mi input; a1 output; rho_vec_I input; e1 output; i1 output; Ohm1 output; omega1 output; f1 output; u1 output; L1 output; l1 output; omega_t1 output; lambda1 output; theta1 output; rho_dot_vec_I input; r0_vec_I input; v0_vec_I input; r1_vec_I output; r1x_I output; r1y_I output; r1z_I output; v1_vec_I output
function [a1,e1,i1,Ohm1,omega1,f1,u1,L1,l1,omega_t1,lambda1,theta1,r1_vec_I,r1x_I,r1y_I,r1z_I,v1_vec_I] = fcn(mi,rho_vec_I,rho_dot_vec_I,r0_vec_I,v0_vec_I)

r1_vec_I = rho_vec_I + r0_vec_I;
r1x_I = r1_vec_I(1);
r1y_I = r1_vec_I(2);
r1z_I = r1_vec_I(3);

v1_vec_I = rho_dot_vec_I + v0_vec_I;

[a1,e1,i1,Ohm1,omega1,f1,u1,L1,l1,omega_t1,lambda1,theta1] = orb_elem(mi,r1_vec_I,v1_vec_I);

== matlab function untitled/wrapTo2pi3 ==
  data: u input; y output
function y = fcn(u)

y = wrapTo2Pi(u);

== matlab function untitled/MATLAB Function6 ==
  data: u input; y output
function y = fcn(u)

y = sqrt(u(1)^2 + u(2)^2 + u(3)^2);

== matlab function untitled/MATLAB Function7 ==
  data: x input; rho output
function rho = fcn(x)

X = x(1);
Y = x(2);
Z = x(3);

rho = sqrt(X^2+Y^2+Z^2);

== matlab function untitled/MATLAB Function8 ==
  data: x input; rho output
function rho = fcn(x)

X = x(1);
Y = x(2);
Z = x(3);

rho = sqrt(X^2+Y^2+Z^2);

== matlab function untitled/MATLAB Function9 ==
  data: x input; rho output
function rho = fcn(x)

X = x(1);
Y = x(2);
Z = x(3);

rho = sqrt(X^2+Y^2+Z^2);

== matlab function untitled/ElemOrbLider2 ==
  data: mi input; ohm input; theta input; I input; x input; a0 output; y input; z input; x_dot input; y_dot input; z_dot input; e0 output; i0 output; Ohm0 output; omega0 output; f0 output; l0 output; omega_t0 output; lambda0 output; theta0 output; r0x_I output; r0y_I output; r0z_I output; r0_vec_I output; v0_vec_I output; h0_vec_I output; L0 output
function [a0,e0,i0,Ohm0,omega0,f0,l0,omega_t0,lambda0,theta0,r0x_I,r0y_I,r0z_I,r0_vec_I,v0_vec_I,h0_vec_I,L0] = fcn(mi,ohm,theta,I,x,y,z,x_dot,y_dot,z_dot)

[~,T_LVLH_In] = TransInerLVLH(ohm,theta,I);

r0_vec_I = T_LVLH_In*[x y z]';

r0x_I = r0_vec_I(1);
r0y_I = r0_vec_I(2);
r0z_I = r0_vec_I(3);

v0_vec_I = T_LVLH_In*[x_dot y_dot z_dot]';

h0_vec_I = cross(r0_vec_I,v0_vec_I);

[a0,e0,i0,Ohm0,omega0,f0,l0,omega_t0,lambda0,theta0,~] = orb_elem(mi,r0_vec_I,v0_vec_I);

%L0 = wrapTo2Pi(omega0 + Ohm0 + f0);
%L0 = wrapTo2Pi(omega0 + Ohm0);
L0 = wrapTo2Pi(Ohm0);

== matlab function untitled/MATLAB Function14 ==
  data: u input; y output
function y = fcn(u)

y = sqrt(u(1)^2 + u(2)^2 + u(3)^2);

== matlab function untitled/MATLAB Function16 ==
  data: x input; rho output
function rho = fcn(x)

X = x(1);
Y = x(2);
Z = x(3);

rho = sqrt(X^2+Y^2+Z^2);

== matlab function untitled/MATLAB Function10 ==
  data: x input; rho output
function rho = fcn(x)

X = x(1);
Y = x(2);
Z = x(3);

rho = sqrt(X^2+Y^2+Z^2);

== matlab function untitled/MATLAB Function17 ==
  data: x input; rho output
function rho = fcn(x)

X = x(1);
Y = x(2);
Z = x(3);

rho = sqrt(X^2+Y^2+Z^2);

== matlab function untitled/MATLAB Function15 ==
  data: u input; y output
function y = fcn(u)

y = sqrt(u(1)^2 + u(2)^2 + u(3)^2);

== matlab function untitled/wrapTo2pi4 ==
  data: u input; y output
function y = fcn(u)

y = wrapTo2Pi(u);

== matlab function untitled/MATLAB Function11 ==
  data: u input; y output
function y = fcn(u)

y = sqrt(u(1)^2 + u(2)^2 + u(3)^2);

== matlab function untitled/MATLAB Function12 ==
  data: C output; r0_vec_I input; h0_vec_I input
function C  = fcn(r0_vec_I,h0_vec_I)

r0_vec_I_uni = r0_vec_I/norm(r0_vec_I);
h0_vec_I_uni = h0_vec_I/norm(h0_vec_I);

ex_vec_uni = r0_vec_I_uni;
ez_vec_uni = h0_vec_I_uni;
ey_vec_uni = cross(ez_vec_uni,ex_vec_uni);

C = [ex_vec_uni(1) ex_vec_uni(2) ex_vec_uni(3)
    ey_vec_uni(1) ey_vec_uni(2) ey_vec_uni(3)
    ez_vec_uni(1) ez_vec_uni(2) ez_vec_uni(3)];

== matlab function untitled/Nadir1 ==
  data: Re input; r0 input; x input; y input; z input; ohm0 input; i0 input; L0 input; ohm1 input; i1 input; L1 input; LF1 output; LF2 output; alpha_F1 output; alpha_F2 output; alpha_f output; PHI output; THETA output; psi_ref output; phi_ref output
function [LF1,LF2,alpha_F1,alpha_F2,alpha_f,PHI,THETA,psi_ref,phi_ref]  = fcn(Re,r0,x,y,z,ohm0,i0,L0,ohm1,i1,L1)

ohm_f = ohm1;
i_f = i1;
ohm_l = ohm0;
i_l = i0;
u0_l = L0;
u0_f = L1;


% Ângulos alpha_f e alpha_l

LF1 = asin(sin(u0_f)*sin(i_f));

if u0_f >=0 && u0_f < pi
    %alpha_F1 = real(acos(complex(cos(u0_f)/cos(LF1))));
    alpha_F1 = (acos((cos(u0_f)/cos(LF1))));
else
    %alpha_F1 = 2*pi - real(acos(complex(cos(u0_f)/cos(LF1))));
    alpha_F1 = 2*pi - (acos((cos(u0_f)/cos(LF1))));
end

alpha_F2 = alpha_F1 + ohm_f;

LF2 = atan(sin(alpha_F2)*tan(i_l));

if u0_f >=0 && u0_f < pi
    alpha_f = acos(cos(LF2)*cos(alpha_F2));
else
    alpha_f = 2*pi - acos(cos(LF2)*cos(alpha_F2));
end

alpha_l = u0_l;

PHI = LF1 - LF2;
THETA = alpha_l - alpha_f;

%% EL (psi)

[~,~,R3_Ohm_l_neg] = transfer(-ohm_l);
[R1_i_l_neg,~,~] = transfer(-i_l);
[~,~,R3_alpha_f_neg] = transfer(-alpha_f);
OA = R3_Ohm_l_neg*R1_i_l_neg*R3_alpha_f_neg*[Re; 0; 0];

[~,~,R3_alpha_l_neg] = transfer(-alpha_l);
FO = -R3_Ohm_l_neg*R1_i_l_neg*R3_alpha_l_neg*[r0+x; y; z];

FA = FO + OA;

if alpha_f >= 0 && alpha_f < pi
    EL = -acos((dot(FA,FO))/(norm(FA)*norm(FO)));
else
    EL = acos((dot(FA,FO))/(norm(FA)*norm(FO)));
end

psi_ref = EL;

%% AZ (phi)

ONL = R3_Ohm_l_neg*R1_i_l_neg*R3_alpha_l_neg*[Re; 0; 0];

FNL = FO + ONL;

AZ = acos((dot(FA,FNL))/(norm(FA)*norm(FNL)));

phi_ref = AZ;

%% Cálculo das matrizes de transferência
    function [T1,T2,T3] = transfer(alpha)
        T1 = [1 0 0; 0 cos(alpha) sin(alpha); 0 -sin(alpha) cos(alpha)];
        T2 = [cos(alpha) 0 -sin(alpha); 0 1 0; sin(alpha) 0 cos(alpha)];
        T3 = [cos(alpha) sin(alpha) 0; -sin(alpha) cos(alpha) 0; 0 0 1];
    end

end

== matlab function untitled/MATLAB Function13 ==
  data: u input; y output
function y = fcn(u)

y = sqrt(u(1)^2 + u(2)^2 + u(3)^2);

== matlab function untitled/MATLAB Function18 ==
  data: x input; rho output
function rho = fcn(x)

X = x(1);
Y = x(2);
Z = x(3);

rho = sqrt(X^2+Y^2+Z^2);

== matlab function untitled/MATLAB Function19 ==
  data: x input; rho output
function rho = fcn(x)

X = x(1);
Y = x(2);
Z = x(3);

rho = sqrt(X^2+Y^2+Z^2);

== matlab function untitled/MATLAB Function4 ==
  data: C input; r1_vec_I output; x input; y input; z input; x_dot input; y_dot input; z_dot input; r0_vec_I input; v0_vec_I input; v1_vec_I output; r1x_vec_I output; r1y_vec_I output; r1z_vec_I output
function [r1_vec_I,v1_vec_I,r1x_vec_I,r1y_vec_I,r1z_vec_I] = fcn(C,x,y,z,x_dot,y_dot,z_dot,r0_vec_I,v0_vec_I)

rho_vec = [x y z]';
rho_dot_vec = [x_dot y_dot z_dot]';

rho_vec_I = C'*rho_vec;
rho_dot_vec_I = C'*rho_dot_vec;

omega_I = cross(r0_vec_I,v0_vec_I)/norm(r0_vec_I)^2;

r1_vec_I = r0_vec_I + rho_vec_I;
v1_vec_I = v0_vec_I + rho_dot_vec_I + cross(omega_I,rho_vec_I);

r1x_vec_I = r1_vec_I(1);
r1y_vec_I = r1_vec_I(2);
r1z_vec_I = r1_vec_I(3);

== matlab function untitled/Nadir3 ==
  data: Re input; r0 input; x input; y input; z input; ohm0 input; i0 input; L0 input; ohm1 input; i1 input; L1 input; AZ output; EL output
function [AZ,EL]  = fcn(Re,r0,x,y,z,ohm0,i0,L0,ohm1,i1,L1)

theta0 = L0;
theta1 = L1;

[~,~,T3Ohm0Neg] = transfer(-ohm0);
[T1i0Neg,~,~] = transfer(-i0);
[~,~,T3theta0Neg] = transfer(-theta0);

FO = -T3Ohm0Neg*T1i0Neg*T3theta0Neg*[r0+x;y;z];
ONl = T3Ohm0Neg*T1i0Neg*T3theta0Neg*[Re;0;0];
FNl = FO + ONl;

[~,~,T3Ohm1Neg] = transfer(-ohm1);
[T1i1Neg,~,~] = transfer(-i1);
[~,~,T3theta1Neg] = transfer(-theta1);
[T1pi_2,~,~] = transfer(pi/2);
[~,T2pi_2,~] = transfer(pi/2);

Fx = T3Ohm1Neg*T1i1Neg*T3theta1Neg*T1pi_2*T2pi_2*[1;0;0];

Fx2 = (cross(FNl,FO))/(norm(cross(FNl,FO)));

AZ = acos(dot(Fx,Fx2)/(norm(Fx)*norm(Fx2)));

if theta0 >= 0 && theta0 < pi
    EL = -acos(dot(FNl,FO)/(norm(FNl)*norm(FO)));
elseif theta0 >= pi && theta0 <= 2*pi
    EL = acos(dot(FNl,FO)/(norm(FNl)*norm(FO)));
else
    EL = 0;
end


% FL = -trans_T3(-ohm0)*trans_T1(-i0)*trans_T3(-theta0)*[x;y;z];
% Fx2 = (cross(FL,FO))/(norm(cross(FL,FO)));
% theta_ref = acos((dot(Fx,Fx2))/(dot(norm(Fx),norm(Fx2))));
% phi_ref = acos((dot(FL,FO))/(dot(norm(FL),norm(FO))));

% if theta0 >= 0 && theta0 < pi
%     phi_ref = -acos((dot(FL,FO))/(dot(norm(FL),norm(FO))));
% elseif theta0 >= pi && theta0 <= 2*pi
%     phi_ref = acos((dot(FL,FO))/(dot(norm(FL),norm(FO))));
% end


% % Ângulos alpha_f e alpha_l
% 
% LF1 = asin(sin(u0_f)*sin(i_f));
% 
% if u0_f >=0 && u0_f < pi
%     %alpha_F1 = real(acos(complex(cos(u0_f)/cos(LF1))));
%     alpha_F1 = (acos((cos(u0_f)/cos(LF1))));
% else
%     %alpha_F1 = 2*pi - real(acos(complex(cos(u0_f)/cos(LF1))));
%     alpha_F1 = 2*pi - (acos((cos(u0_f)/cos(LF1))));
% end
% 
% alpha_F2 = alpha_F1 + ohm_f;
% 
% LF2 = atan(sin(alpha_F2)*tan(i_l));
% 
% if u0_f >=0 && u0_f < pi
%     alpha_f = acos(cos(LF2)*cos(alpha_F2));
% else
%     alpha_f = 2*pi - acos(cos(LF2)*cos(alpha_F2));
% end
% 
% alpha_l = u0_l;
% 
% PHI = LF1 - LF2;
% THETA = alpha_l - alpha_f;
% 
% %% EL (psi)
% 
% [~,~,R3_Ohm_l_neg] = transfer(-ohm_l);
% [R1_i_l_neg,~,~] = transfer(-i_l);
% [~,~,R3_alpha_f_neg] = transfer(-alpha_f);
% OA = R3_Ohm_l_neg*R1_i_l_neg*R3_alpha_f_neg*[Re; 0; 0];
% 
% [~,~,R3_alpha_l_neg] = transfer(-alpha_l);
% FO = -R3_Ohm_l_neg*R1_i_l_neg*R3_alpha_l_neg*[r0+x; y; z];
% 
% FA = FO + OA;
% 
% if alpha_f >= 0 && alpha_f < pi
%     EL = -acos((dot(FA,FO))/(norm(FA)*norm(FO)));
% else
%     EL = acos((dot(FA,FO))/(norm(FA)*norm(FO)));
% end
% 
% psi_ref = EL;
% 
% %% AZ (phi)
% 
% ONL = R3_Ohm_l_neg*R1_i_l_neg*R3_alpha_l_neg*[Re; 0; 0];
% 
% FNL = FO + ONL;
% 
% AZ = acos((dot(FA,FNL))/(norm(FA)*norm(FNL)));
% 
% phi_ref = AZ;

%% Cálculo das matrizes de transferência
    function [T1,T2,T3] = transfer(alpha)
        T1 = [1 0 0; 0 cos(alpha) sin(alpha); 0 -sin(alpha) cos(alpha)];
        T2 = [cos(alpha) 0 -sin(alpha); 0 1 0; sin(alpha) 0 cos(alpha)];
        T3 = [cos(alpha) sin(alpha) 0; -sin(alpha) cos(alpha) 0; 0 0 1];
    end

end

== matlab function untitled/wrapTo2pi5 ==
  data: u input; y output
function y = fcn(u)

y = wrapTo2Pi(u);

== matlab function untitled/wrapTo2pi6 ==
  data: u input; y output
function y = fcn(u)

y = wrapTo2Pi(u);
